simulink model "testTop"  (R2023b)
settings: Solver=VariableStepAuto  StartTime=0.0  StopTime=10  RelTol=1e-3
PreLoadFcn:
  | slBus1 = Simulink.Bus;
  | slBus1.Description = '';
  | slBus1.DataScope = 'Auto';
  | slBus1.HeaderFile = '';
  | slBus1.Alignment = -1;
  | slBus1.PreserveElementDimensions = false;
  | saveVarsTmp{1} = Simulink.BusElement;
  | saveVarsTmp{1}.Name = 'a';
  | saveVarsTmp{1}.Complexity = 'real';
  | saveVarsTmp{1}.Dimensions = [1 1];
  | saveVarsTmp{1}.DataType = 'double';
  | saveVarsTmp{1}.Min = [];
  | saveVarsTmp{1}.Max = [];
  | saveVarsTmp{1}.DimensionsMode = 'Fixed';
  | saveVarsTmp{1}.SamplingMode = 'Sample based';
  | saveVarsTmp{1}.DocUnits = '';
  | saveVarsTmp{1}.Description = '';
  | saveVarsTmp{1}(2, 1) = Simulink.BusElement;
  | saveVarsTmp{1}(2, 1).Name = 'b';
  | saveVarsTmp{1}(2, 1).Complexity = 'real';
  | saveVarsTmp{1}(2, 1).Dimensions = [1 1];
  | saveVarsTmp{1}(2, 1).DataType = 'double';
  | saveVarsTmp{1}(2, 1).Min = [];
  | saveVarsTmp{1}(2, 1).Max = [];
  | saveVarsTmp{1}(2, 1).DimensionsMode = 'Fixed';
  | saveVarsTmp{1}(2, 1).SamplingMode = 'Sample based';
  | saveVarsTmp{1}(2, 1).DocUnits = '';
  | saveVarsTmp{1}(2, 1).Description = '';
  | slBus1.Elements = saveVarsTmp{1};
  | clear saveVarsTmp;
  | 
  | 
  | u = timeseries([0 1],[0 5]);
values from neighbouring files (symbols this model uses):
  s = 2.0    [busesDD.sldd]
settings Model: DataDictionary=busesDD.sldd  Creator=grouleau  LastModifiedBy=guirl

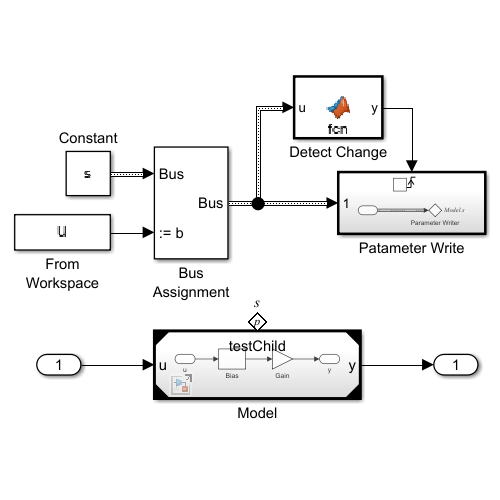
[thumbnail: Simulink's stored preview of the top-level diagram]
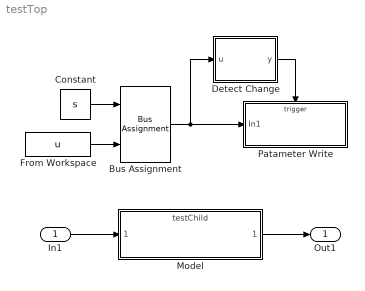
== system testTop ==
  In1 : Inport
  Bus Assignment : BusAssignment  AssignedSignals=b
  Constant : Constant  Value=s  OutDataTypeStr=Bus: slBus1
  Detect Change : MATLAB Function  TreatAsAtomicUnit=on
  From Workspace : FromWorkspace  VariableName=u  SampleTime=0.1  Interpolate=off  OutputAfterFinalValue=Holding final value
  Model : ModelReference  ModelNameDialog=testChild  UsingDefaultArgumentValue=0  ModelReferenceVersion=1.7
  Patameter Write : Subsystem  TreatAsAtomicUnit=on
  Out1 : Outport
  wires:
  In1/1 -> Model/1
  Model/1 -> Out1/1
  Constant/1 -> Bus Assignment/1
  From Workspace/1 -> Bus Assignment/2
  Bus Assignment/1 -> Patameter Write/1(In1), Detect Change/1(u)
  Detect Change/1(y) -> Patameter Write/Trigger

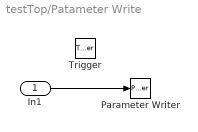
== system testTop/Patameter Write ==
  In1 : Inport
  Trigger : TriggerPort  VariantControl=(inherit)
  Parameter Writer : ParameterWriter  ParameterOwnerBlock=../../Model  ParameterName=s  ParameterInternalName=s
  wires:
  In1/1 -> Parameter Writer/1

== matlab function testTop/Detect Change ==
  data: u input Bus: slBus1; y output
function y = fcn(u)
persistent u_previous
if isempty(u_previous)
    u_previous = u;
end
y = isequal(u,u_previous);
u_previous = u;
